simulink model "modelloForKalman"  (R2019a)
settings: Solver=ode8  StartTime=0.0  StopTime=(N-1)*Ts  FixedStep=Ts  RelTol=1e-3
values from neighbouring files (symbols this model uses):
  b = 0.50    (= 0.5)    [ExtendedKalmanFilter.m]    (also in f.m = x(2,k)-((g*Ts)/L)*sin(x(1,k))-((b*Ts)/(m*L))*x(2,k)+(Ts/(m*L; generaMatriceF.m = 1-((b*Ts)/(m*L)); main.m)
  g = 9.81    [ExtendedKalmanFilter.m]    (also in main.m)
  I = eye(2)    [ExtendedKalmanFilter.m]    (also in main.m = 0.088)
  L = 0.40    (= 0.4)    [ExtendedKalmanFilter.m]    (also in main.m)
  m = 0.55    [ExtendedKalmanFilter.m]    (also in main.m)
  Ts = 0.05    [ExtendedKalmanFilter.m]    (also in main.m)
settings Model: Creator=39338  LastModifiedBy=39338
settings DataIOCC: SaveOutput=off  SignalLogging=off  DSMLogging=off  SaveTime=off  ReturnWorkspaceOutputs=off

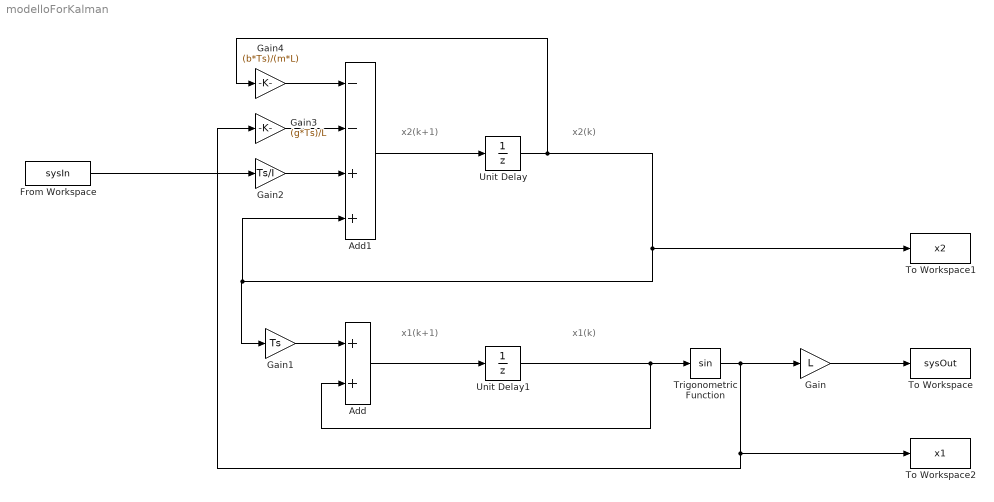
== system modelloForKalman ==
  note: x2(k)
  note: x1(k+1)
  note: x1(k)
  note: x2(k+1)
  Add : Sum
  Add1 : Sum  Inputs=--++
  From Workspace : FromWorkspace  VariableName=sysIn  SampleTime=Ts
  Gain : Gain  Gain=L
  Gain1 : Gain  Gain=Ts
  Gain2 : Gain  Gain=Ts/I
  Gain3 : Gain  Gain=(g*Ts)/L
  Gain4 : Gain  Gain=(b*Ts)/(m*L)
  To Workspace : ToWorkspace  VariableName=sysOut  SampleTime=Ts
      settings: Save2DSignal=2-D array (concatenate along first dimension)
  To Workspace1 : ToWorkspace  VariableName=x2  SampleTime=Ts
      settings: Save2DSignal=2-D array (concatenate along first dimension)
  To Workspace2 : ToWorkspace  VariableName=x1  SampleTime=Ts
      settings: Save2DSignal=2-D array (concatenate along first dimension)
  Trigonometric Function : Trigonometry
  Unit Delay : UnitDelay  SampleTime=Ts  HasFrameUpgradeWarning=on
  Unit Delay1 : UnitDelay  SampleTime=Ts  HasFrameUpgradeWarning=on
  wires:
  From Workspace/1 -> Gain2/1
  Trigonometric Function/1 -> Gain3/1, To Workspace2/1, Gain/1
  Gain4/1 -> Add1/1
  Gain2/1 -> Add1/3
  Add1/1 -> Unit Delay/1
  Gain3/1 -> Add1/2
  Gain1/1 -> Add/1
  Gain/1 -> To Workspace/1
  Unit Delay1/1 -> Add/2, Trigonometric Function/1
  Add/1 -> Unit Delay1/1
  Unit Delay/1 -> Gain4/1, To Workspace1/1, Add1/4, Gain1/1
